simulink model "n_vector"  (R2016b)
settings: Solver=VariableStepAuto  StartTime=0.0  StopTime=10.0  RelTol=1e-3
values from neighbouring files (symbols this model uses):
  F = [0.1, 0 ... (first row only)    [parameters.m]
settings Model: Creator=kma  LastModifiedBy=kma

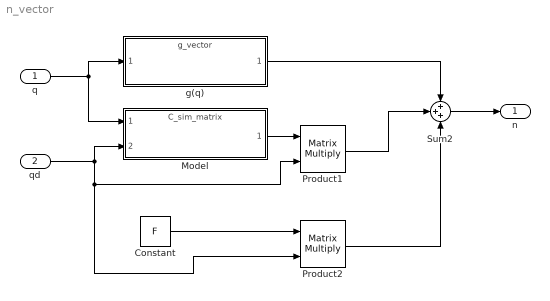
== system n_vector ==
  q : Inport  PortDimensions=2
  qd : Inport  Port=2  PortDimensions=2
  Constant : Constant  Value=F
  Model : ModelReference  ModelNameDialog=C_sim_matrix.slx  SimulationMode=Normal  ModelReferenceVersion=1.2
  Product1 : Product  Multiplication=Matrix(*)
  Product2 : Product  Multiplication=Matrix(*)
  Sum2 : Sum  Inputs=+++
  g(q) : ModelReference  ModelNameDialog=g_vector.slx  SimulationMode=Normal  ModelReferenceVersion=1.8
  n : Outport
  wires:
  Constant/1 -> Product2/1
  qd/1 -> Model/2, Product1/2, Product2/2
  Model/1 -> Product1/1
  q/1 -> Model/1, g(q)/1
  g(q)/1 -> Sum2/1
  Product1/1 -> Sum2/2
  Product2/1 -> Sum2/3
  Sum2/1 -> n/1
